simulink subsystem "RoboticArmViperX300"  (R2022a)
settings: Solver=VariableStepAuto  StartTime=0.0  StopTime=10.0  RelTol=1e-3
undefined symbols (not defined in the file or in its folder): smiData, X, Y, Z
libraries: sm_lib x102, nesl_utility x58
(part 1 of 3)
settings Model: Creator=Andy  LastModifiedBy=Andy

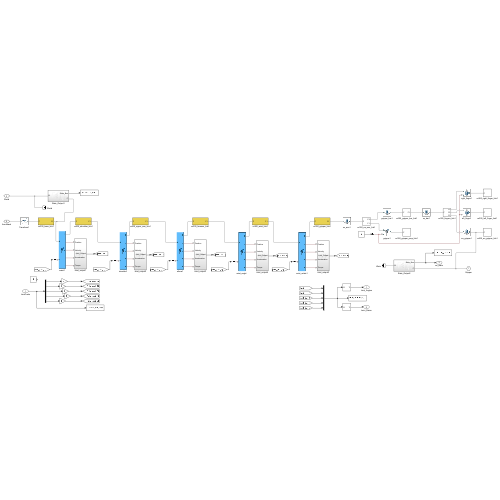
[thumbnail: Simulink's stored preview of the top-level diagram]
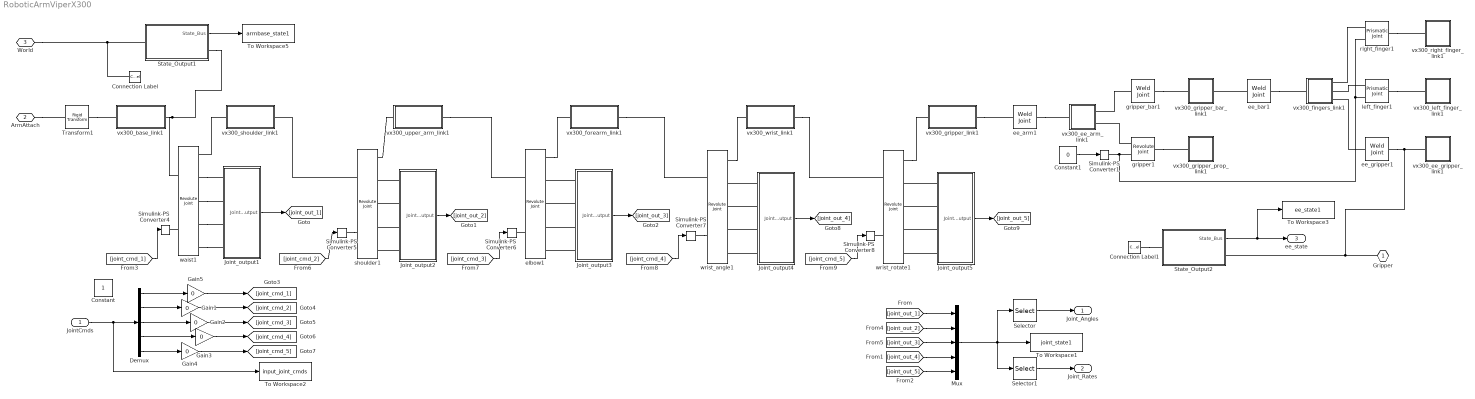
== system RoboticArmViperX300 ==
  JointCmds : Inport
  Connection Label : ConnectionLabel  Label=World
  Connection Label1 : ConnectionLabel  Label=World
  Constant : Constant
  Constant1 : Constant  Value=0
  Demux : Demux  Outputs=5
  Gain{1..5} (5 alike) : Gain  Gain=0
  Joint_output1 : Subsystem
  Joint_output2 : Subsystem
  Joint_output3 : Subsystem
  Joint_output4 : Subsystem
  Joint_output5 : Subsystem
  Mux : Mux  Inputs=5
  Selector : Selector  InputPortWidth=20  IndexOptions=Index vector (dialog)  Indices=[1 5 9 13 17]  OutputSizes=1
  Selector1 : Selector  InputPortWidth=20  IndexOptions=Index vector (dialog)  Indices=[2 6 10 14 18]  OutputSizes=1
  Simulink-PS Converter{1,4..8} (6 alike) : nesl_utility/Simulink-PS Converter  PhysicalDomain=network_engine_domain  SubClassName=ps_input  LeftPortType=input  RightPortType=output  PseudoPeriodic=off  Frequencies=[]  NoiseDistribution=none  NoiseParameters=[]  Unit=1  AffineConversion=off  FilteringAndDerivatives=filter  SimscapeFilterOrder=2  InputFilterTimeConstant=0.001  UdotUserProvided=0
      settings: SourceProductBaseCode=SS,PW,VE
  State_Output1 : Subsystem
  State_Output2 : Subsystem
  To Workspace1 : ToWorkspace  VariableName=joint_state1  SaveFormat=Timeseries  SampleTime=-1
  To Workspace2 : ToWorkspace  VariableName=input_joint_cmds  SaveFormat=Timeseries  SampleTime=-1
  To Workspace3 : ToWorkspace  VariableName=ee_state1  SaveFormat=Timeseries  SampleTime=-1
  To Workspace5 : ToWorkspace  VariableName=armbase_state1  SaveFormat=Timeseries  SampleTime=-1
  Transform1 : sm_lib/Frames and Transforms/Rigid Transform  TranslationMethod=Cartesian  TranslationStandardOffset=0  TranslationLengthUnit=mm  TranslationStandardAxis=+Z  TranslationCartesianOffset=smiData.RigidTransform(1).translation  TranslationROffset=0  TranslationROffsetUnits=m  TranslationZOffset=0  TranslationZOffsetUnits=m  TranslationThetaOffset=0  TranslationThetaOffsetUnits=deg  RotationMethod=ArbitraryAxis  RotationAngleUnits=rad  RotationStandardAxis=+Z  RotationAngle=smiData.RigidTransform(1).angle  RotationArbitraryAxis=smiData.RigidTransform(1).axis  FollAlignAxisA=+X  BaseAlignAxisA=+Y  FollAlignAxisB=+Y  BaseAlignAxisB=+Z  RotationSequenceAxes=FollowerAxes  RotationSequence=YZX  RotationSequenceAngles=[0 0 0]  RotationSequenceAnglesUnits=deg  RotationMatrix=[1 0 0; 0 1 0; 0 0 1]
  ee_arm1 : sm_lib/Joints/Weld Joint  JointMode=Normal  SenseConstraintForce=off  SenseConstraintForceX=off  SenseConstraintForceY=off  SenseConstraintForceZ=off  SenseConstraintTorque=off  SenseConstraintTorqueX=off  SenseConstraintTorqueY=off  SenseConstraintTorqueZ=off  SenseTotalForce=off  SenseTotalForceX=off  SenseTotalForceY=off  SenseTotalForceZ=off  SenseTotalTorque=off  SenseTotalTorqueX=off  SenseTotalTorqueY=off  SenseTotalTorqueZ=off  CompositeWrenchDir=FollowerOnBase  CompositeWrenchFrame=BaseFrame
  ee_bar1 : sm_lib/Joints/Weld Joint  JointMode=Normal  SenseConstraintForce=off  SenseConstraintForceX=off  SenseConstraintForceY=off  SenseConstraintForceZ=off  SenseConstraintTorque=off  SenseConstraintTorqueX=off  SenseConstraintTorqueY=off  SenseConstraintTorqueZ=off  SenseTotalForce=off  SenseTotalForceX=off  SenseTotalForceY=off  SenseTotalForceZ=off  SenseTotalTorque=off  SenseTotalTorqueX=off  SenseTotalTorqueY=off  SenseTotalTorqueZ=off  CompositeWrenchDir=FollowerOnBase  CompositeWrenchFrame=BaseFrame
  ee_gripper1 : sm_lib/Joints/Weld Joint  JointMode=Normal  SenseConstraintForce=off  SenseConstraintForceX=off  SenseConstraintForceY=off  SenseConstraintForceZ=off  SenseConstraintTorque=off  SenseConstraintTorqueX=off  SenseConstraintTorqueY=off  SenseConstraintTorqueZ=off  SenseTotalForce=off  SenseTotalForceX=off  SenseTotalForceY=off  SenseTotalForceZ=off  SenseTotalTorque=off  SenseTotalTorqueX=off  SenseTotalTorqueY=off  SenseTotalTorqueZ=off  CompositeWrenchDir=FollowerOnBase  CompositeWrenchFrame=BaseFrame
  elbow1 : sm_lib/Joints/Revolute Joint  JointMode=Normal  SenseConstraintForce=off  SenseConstraintForceX=off  SenseConstraintForceY=off  SenseConstraintForceZ=off  SenseConstraintTorque=off  SenseConstraintTorqueX=off  SenseConstraintTorqueY=off  SenseConstraintTorqueZ=off  SenseTotalForce=off  SenseTotalForceX=off  SenseTotalForceY=off  SenseTotalForceZ=off  SenseTotalTorque=on  SenseTotalTorqueX=off  SenseTotalTorqueY=off  SenseTotalTorqueZ=off  CompositeWrenchDir=FollowerOnBase  CompositeWrenchFrame=BaseFrame  EquilibriumPosition=0  EquilibriumPositionUnits=deg  SpringStiffness=0  SpringStiffnessUnits=N*m/deg  DampingCoefficient=0  DampingCoefficientUnits=kg*m^2/(rad*s)  TorqueActuationMode=InputTorque  MotionActuationMode=ComputedMotion  SensePosition=on  SenseVelocity=on  SenseAcceleration=on  SenseTorqueForce=off  SenseLowerLimitTorqueForce=off  SenseUpperLimitTorqueForce=off  LowerLimitSpecify=on  LowerLimitBound=-1.762782544514273  LowerLimitBoundUnits=rad  LowerLimitStiffness=1e4  LowerLimitStiffnessUnits=N*m/deg  LowerLimitDamping=10  LowerLimitDampingUnits=N*m/(deg/s)  LowerLimitTransitionRegionWidth=0.1  LowerLimitTransitionRegionWidthUnits=deg  UpperLimitSpecify=on  UpperLimitBound=1.605702911834783  UpperLimitBoundUnits=rad  UpperLimitStiffness=1e4  UpperLimitStiffnessUnits=N*m/deg  UpperLimitDamping=10  UpperLimitDampingUnits=N*m/(deg/s)  UpperLimitTransitionRegionWidth=0.1  UpperLimitTransitionRegionWidthUnits=deg  PositionTargetSpecify=on  PositionTargetPriority=High  PositionTargetValue=smiData.RevoluteJoint(3).Rz.Pos  PositionTargetValueUnits=deg  VelocityTargetSpecify=off  VelocityTargetPriority=High  VelocityTargetValue=0  VelocityTargetValueUnits=deg/s
  gripper1 : sm_lib/Joints/Revolute Joint  JointMode=Normal  SenseConstraintForce=off  SenseConstraintForceX=off  SenseConstraintForceY=off  SenseConstraintForceZ=off  SenseConstraintTorque=off  SenseConstraintTorqueX=off  SenseConstraintTorqueY=off  SenseConstraintTorqueZ=off  SenseTotalForce=off  SenseTotalForceX=off  SenseTotalForceY=off  SenseTotalForceZ=off  SenseTotalTorque=off  SenseTotalTorqueX=off  SenseTotalTorqueY=off  SenseTotalTorqueZ=off  CompositeWrenchDir=FollowerOnBase  CompositeWrenchFrame=BaseFrame  EquilibriumPosition=0  EquilibriumPositionUnits=deg  SpringStiffness=0  SpringStiffnessUnits=N*m/deg  DampingCoefficient=0  DampingCoefficientUnits=kg*m^2/(rad*s)  TorqueActuationMode=ComputedTorque  MotionActuationMode=InputMotion  SensePosition=off  SenseVelocity=off  SenseAcceleration=off  SenseTorqueForce=off  SenseLowerLimitTorqueForce=off  SenseUpperLimitTorqueForce=off  LowerLimitSpecify=off  LowerLimitBound=-90  LowerLimitBoundUnits=deg  LowerLimitStiffness=1e4  LowerLimitStiffnessUnits=N*m/deg  LowerLimitDamping=10  LowerLimitDampingUnits=N*m/(deg/s)  LowerLimitTransitionRegionWidth=0.1  LowerLimitTransitionRegionWidthUnits=deg  UpperLimitSpecify=off  UpperLimitBound=90  UpperLimitBoundUnits=deg  UpperLimitStiffness=1e4  UpperLimitStiffnessUnits=N*m/deg  UpperLimitDamping=10  UpperLimitDampingUnits=N*m/(deg/s)  UpperLimitTransitionRegionWidth=0.1  UpperLimitTransitionRegionWidthUnits=deg  PositionTargetSpecify=off  PositionTargetPriority=High  PositionTargetValue=0  PositionTargetValueUnits=deg  VelocityTargetSpecify=off  VelocityTargetPriority=High  VelocityTargetValue=0  VelocityTargetValueUnits=deg/s
  gripper_bar1 : sm_lib/Joints/Weld Joint  JointMode=Normal  SenseConstraintForce=off  SenseConstraintForceX=off  SenseConstraintForceY=off  SenseConstraintForceZ=off  SenseConstraintTorque=off  SenseConstraintTorqueX=off  SenseConstraintTorqueY=off  SenseConstraintTorqueZ=off  SenseTotalForce=off  SenseTotalForceX=off  SenseTotalForceY=off  SenseTotalForceZ=off  SenseTotalTorque=off  SenseTotalTorqueX=off  SenseTotalTorqueY=off  SenseTotalTorqueZ=off  CompositeWrenchDir=FollowerOnBase  CompositeWrenchFrame=BaseFrame
  left_finger1 : sm_lib/Joints/Prismatic Joint  JointMode=Normal  SenseConstraintForce=off  SenseConstraintForceX=off  SenseConstraintForceY=off  SenseConstraintForceZ=off  SenseConstraintTorque=off  SenseConstraintTorqueX=off  SenseConstraintTorqueY=off  SenseConstraintTorqueZ=off  SenseTotalForce=off  SenseTotalForceX=off  SenseTotalForceY=off  SenseTotalForceZ=off  SenseTotalTorque=off  SenseTotalTorqueX=off  SenseTotalTorqueY=off  SenseTotalTorqueZ=off  CompositeWrenchDir=FollowerOnBase  CompositeWrenchFrame=BaseFrame  EquilibriumPosition=0  EquilibriumPositionUnits=m  SpringStiffness=0  SpringStiffnessUnits=N/m  DampingCoefficient=0  DampingCoefficientUnits=kg/s  TorqueActuationMode=ComputedTorque  MotionActuationMode=InputMotion  SensePosition=off  SenseVelocity=off  SenseAcceleration=off  SenseTorqueForce=off  SenseLowerLimitTorqueForce=off  SenseUpperLimitTorqueForce=off  LowerLimitSpecify=on  LowerLimitBound=0.021  LowerLimitBoundUnits=m  LowerLimitStiffness=1e6  LowerLimitStiffnessUnits=N/m  LowerLimitDamping=1e3  LowerLimitDampingUnits=N/(m/s)  LowerLimitTransitionRegionWidth=1e-4  LowerLimitTransitionRegionWidthUnits=m  UpperLimitSpecify=on  UpperLimitBound=0.057  UpperLimitBoundUnits=m  UpperLimitStiffness=1e6  UpperLimitStiffnessUnits=N/m  UpperLimitDamping=1e3  UpperLimitDampingUnits=N/(m/s)  UpperLimitTransitionRegionWidth=1e-4  UpperLimitTransitionRegionWidthUnits=m  PositionTargetSpecify=off  PositionTargetPriority=High  PositionTargetValue=0  PositionTargetValueUnits=m  VelocityTargetSpecify=off  VelocityTargetPriority=High  VelocityTargetValue=0  VelocityTargetValueUnits=m/s
  right_finger1 : sm_lib/Joints/Prismatic Joint  JointMode=Normal  SenseConstraintForce=off  SenseConstraintForceX=off  SenseConstraintForceY=off  SenseConstraintForceZ=off  SenseConstraintTorque=off  SenseConstraintTorqueX=off  SenseConstraintTorqueY=off  SenseConstraintTorqueZ=off  SenseTotalForce=off  SenseTotalForceX=off  SenseTotalForceY=off  SenseTotalForceZ=off  SenseTotalTorque=off  SenseTotalTorqueX=off  SenseTotalTorqueY=off  SenseTotalTorqueZ=off  CompositeWrenchDir=FollowerOnBase  CompositeWrenchFrame=BaseFrame  EquilibriumPosition=0  EquilibriumPositionUnits=m  SpringStiffness=0  SpringStiffnessUnits=N/m  DampingCoefficient=0  DampingCoefficientUnits=kg/s  TorqueActuationMode=ComputedTorque  MotionActuationMode=InputMotion  SensePosition=off  SenseVelocity=off  SenseAcceleration=off  SenseTorqueForce=off  SenseLowerLimitTorqueForce=off  SenseUpperLimitTorqueForce=off  LowerLimitSpecify=on  LowerLimitBound=-0.057  LowerLimitBoundUnits=m  LowerLimitStiffness=1e6  LowerLimitStiffnessUnits=N/m  LowerLimitDamping=1e3  LowerLimitDampingUnits=N/(m/s)  LowerLimitTransitionRegionWidth=1e-4  LowerLimitTransitionRegionWidthUnits=m  UpperLimitSpecify=on  UpperLimitBound=-0.021  UpperLimitBoundUnits=m  UpperLimitStiffness=1e6  UpperLimitStiffnessUnits=N/m  UpperLimitDamping=1e3  UpperLimitDampingUnits=N/(m/s)  UpperLimitTransitionRegionWidth=1e-4  UpperLimitTransitionRegionWidthUnits=m  PositionTargetSpecify=off  PositionTargetPriority=High  PositionTargetValue=0  PositionTargetValueUnits=m  VelocityTargetSpecify=off  VelocityTargetPriority=High  VelocityTargetValue=0  VelocityTargetValueUnits=m/s
  shoulder1 : sm_lib/Joints/Revolute Joint  JointMode=Normal  SenseConstraintForce=off  SenseConstraintForceX=off  SenseConstraintForceY=off  SenseConstraintForceZ=off  SenseConstraintTorque=off  SenseConstraintTorqueX=off  SenseConstraintTorqueY=off  SenseConstraintTorqueZ=off  SenseTotalForce=off  SenseTotalForceX=off  SenseTotalForceY=off  SenseTotalForceZ=off  SenseTotalTorque=on  SenseTotalTorqueX=off  SenseTotalTorqueY=off  SenseTotalTorqueZ=off  CompositeWrenchDir=FollowerOnBase  CompositeWrenchFrame=BaseFrame  EquilibriumPosition=0  EquilibriumPositionUnits=deg  SpringStiffness=0  SpringStiffnessUnits=N*m/deg  DampingCoefficient=0  DampingCoefficientUnits=kg*m^2/(rad*s)  TorqueActuationMode=InputTorque  MotionActuationMode=ComputedMotion  SensePosition=on  SenseVelocity=on  SenseAcceleration=on  SenseTorqueForce=off  SenseLowerLimitTorqueForce=off  SenseUpperLimitTorqueForce=off  LowerLimitSpecify=on  LowerLimitBound=-1.850049007113989  LowerLimitBoundUnits=rad  LowerLimitStiffness=1e4  LowerLimitStiffnessUnits=N*m/deg  LowerLimitDamping=10  LowerLimitDampingUnits=N*m/(deg/s)  LowerLimitTransitionRegionWidth=0.1  LowerLimitTransitionRegionWidthUnits=deg  UpperLimitSpecify=on  UpperLimitBound=1.256637061435917  UpperLimitBoundUnits=rad  UpperLimitStiffness=1e4  UpperLimitStiffnessUnits=N*m/deg  UpperLimitDamping=10  UpperLimitDampingUnits=N*m/(deg/s)  UpperLimitTransitionRegionWidth=0.1  UpperLimitTransitionRegionWidthUnits=deg  PositionTargetSpecify=on  PositionTargetPriority=High  PositionTargetValue=smiData.RevoluteJoint(2).Rz.Pos  PositionTargetValueUnits=deg  VelocityTargetSpecify=off  VelocityTargetPriority=High  VelocityTargetValue=0  VelocityTargetValueUnits=deg/s
  vx300_base_link1 : Subsystem
  vx300_ee_arm_link1 : Subsystem
  vx300_ee_gripper_link1 : Subsystem
  vx300_fingers_link1 : Subsystem
  vx300_forearm_link1 : Subsystem
  vx300_gripper_bar_link1 : Subsystem
  vx300_gripper_link1 : Subsystem
  vx300_gripper_prop_link1 : Subsystem
  vx300_left_finger_link1 : Subsystem
  vx300_right_finger_link1 : Subsystem
  vx300_shoulder_link1 : Subsystem
  vx300_upper_arm_link1 : Subsystem
  vx300_wrist_link1 : Subsystem
  waist1 : sm_lib/Joints/Revolute Joint  JointMode=Normal  SenseConstraintForce=off  SenseConstraintForceX=off  SenseConstraintForceY=off  SenseConstraintForceZ=off  SenseConstraintTorque=off  SenseConstraintTorqueX=off  SenseConstraintTorqueY=off  SenseConstraintTorqueZ=off  SenseTotalForce=off  SenseTotalForceX=off  SenseTotalForceY=off  SenseTotalForceZ=off  SenseTotalTorque=on  SenseTotalTorqueX=off  SenseTotalTorqueY=off  SenseTotalTorqueZ=off  CompositeWrenchDir=FollowerOnBase  CompositeWrenchFrame=BaseFrame  EquilibriumPosition=0  EquilibriumPositionUnits=deg  SpringStiffness=0  SpringStiffnessUnits=N*m/deg  DampingCoefficient=0  DampingCoefficientUnits=kg*m^2/(rad*s)  TorqueActuationMode=InputTorque  MotionActuationMode=ComputedMotion  SensePosition=on  SenseVelocity=on  SenseAcceleration=on  SenseTorqueForce=off  SenseLowerLimitTorqueForce=off  SenseUpperLimitTorqueForce=off  LowerLimitSpecify=on  LowerLimitBound=-3.141582653589793  LowerLimitBoundUnits=rad  LowerLimitStiffness=1e4  LowerLimitStiffnessUnits=N*m/deg  LowerLimitDamping=10  LowerLimitDampingUnits=N*m/(deg/s)  LowerLimitTransitionRegionWidth=0.1  LowerLimitTransitionRegionWidthUnits=deg  UpperLimitSpecify=on  UpperLimitBound=3.141582653589793  UpperLimitBoundUnits=rad  UpperLimitStiffness=1e4  UpperLimitStiffnessUnits=N*m/deg  UpperLimitDamping=10  UpperLimitDampingUnits=N*m/(deg/s)  UpperLimitTransitionRegionWidth=0.1  UpperLimitTransitionRegionWidthUnits=deg  PositionTargetSpecify=on  PositionTargetPriority=High  PositionTargetValue=smiData.RevoluteJoint(1).Rz.Pos  PositionTargetValueUnits=deg  VelocityTargetSpecify=off  VelocityTargetPriority=High  VelocityTargetValue=0  VelocityTargetValueUnits=deg/s
  wrist_angle1 : sm_lib/Joints/Revolute Joint  JointMode=Normal  SenseConstraintForce=off  SenseConstraintForceX=off  SenseConstraintForceY=off  SenseConstraintForceZ=off  SenseConstraintTorque=off  SenseConstraintTorqueX=off  SenseConstraintTorqueY=off  SenseConstraintTorqueZ=off  SenseTotalForce=off  SenseTotalForceX=off  SenseTotalForceY=off  SenseTotalForceZ=off  SenseTotalTorque=on  SenseTotalTorqueX=off  SenseTotalTorqueY=off  SenseTotalTorqueZ=off  CompositeWrenchDir=FollowerOnBase  CompositeWrenchFrame=BaseFrame  EquilibriumPosition=0  EquilibriumPositionUnits=deg  SpringStiffness=0  SpringStiffnessUnits=N*m/deg  DampingCoefficient=0  DampingCoefficientUnits=kg*m^2/(rad*s)  TorqueActuationMode=InputTorque  MotionActuationMode=ComputedMotion  SensePosition=on  SenseVelocity=on  SenseAcceleration=on  SenseTorqueForce=off  SenseLowerLimitTorqueForce=off  SenseUpperLimitTorqueForce=off  LowerLimitSpecify=on  LowerLimitBound=-1.867502299633933  LowerLimitBoundUnits=rad  LowerLimitStiffness=1e4  LowerLimitStiffnessUnits=N*m/deg  LowerLimitDamping=10  LowerLimitDampingUnits=N*m/(deg/s)  LowerLimitTransitionRegionWidth=0.1  LowerLimitTransitionRegionWidthUnits=deg  UpperLimitSpecify=on  UpperLimitBound=2.234021442552742  UpperLimitBoundUnits=rad  UpperLimitStiffness=1e4  UpperLimitStiffnessUnits=N*m/deg  UpperLimitDamping=10  UpperLimitDampingUnits=N*m/(deg/s)  UpperLimitTransitionRegionWidth=0.1  UpperLimitTransitionRegionWidthUnits=deg  PositionTargetSpecify=on  PositionTargetPriority=High  PositionTargetValue=smiData.RevoluteJoint(4).Rz.Pos  PositionTargetValueUnits=deg  VelocityTargetSpecify=off  VelocityTargetPriority=High  VelocityTargetValue=0  VelocityTargetValueUnits=deg/s
  wrist_rotate1 : sm_lib/Joints/Revolute Joint  JointMode=Normal  SenseConstraintForce=off  SenseConstraintForceX=off  SenseConstraintForceY=off  SenseConstraintForceZ=off  SenseConstraintTorque=off  SenseConstraintTorqueX=off  SenseConstraintTorqueY=off  SenseConstraintTorqueZ=off  SenseTotalForce=off  SenseTotalForceX=off  SenseTotalForceY=off  SenseTotalForceZ=off  SenseTotalTorque=on  SenseTotalTorqueX=off  SenseTotalTorqueY=off  SenseTotalTorqueZ=off  CompositeWrenchDir=FollowerOnBase  CompositeWrenchFrame=BaseFrame  EquilibriumPosition=0  EquilibriumPositionUnits=deg  SpringStiffness=0  SpringStiffnessUnits=N*m/deg  DampingCoefficient=0  DampingCoefficientUnits=kg*m^2/(rad*s)  TorqueActuationMode=InputTorque  MotionActuationMode=ComputedMotion  SensePosition=on  SenseVelocity=on  SenseAcceleration=on  SenseTorqueForce=off  SenseLowerLimitTorqueForce=off  SenseUpperLimitTorqueForce=off  LowerLimitSpecify=on  LowerLimitBound=-3.141582653589793  LowerLimitBoundUnits=rad  LowerLimitStiffness=1e4  LowerLimitStiffnessUnits=N*m/deg  LowerLimitDamping=10  LowerLimitDampingUnits=N*m/(deg/s)  LowerLimitTransitionRegionWidth=0.1  LowerLimitTransitionRegionWidthUnits=deg  UpperLimitSpecify=on  UpperLimitBound=3.141582653589793  UpperLimitBoundUnits=rad  UpperLimitStiffness=1e4  UpperLimitStiffnessUnits=N*m/deg  UpperLimitDamping=10  UpperLimitDampingUnits=N*m/(deg/s)  UpperLimitTransitionRegionWidth=0.1  UpperLimitTransitionRegionWidthUnits=deg  PositionTargetSpecify=on  PositionTargetPriority=High  PositionTargetValue=smiData.RevoluteJoint(5).Rz.Pos  PositionTargetValueUnits=deg  VelocityTargetSpecify=off  VelocityTargetPriority=High  VelocityTargetValue=0  VelocityTargetValueUnits=deg/s
  Gripper : PMIOPort  Side=Right
  ArmAttach : PMIOPort  Port=2  Side=Left
  World : PMIOPort  Port=3  Side=Left
  Joint_Angles : Outport
  Joint_Rates : Outport  Port=2
  ee_state : Outport  Port=3
  wires:
  Joint_output3/1(Joint_Output) -> [joint_out_3]
  [joint_out_1] -> Mux/1
  Selector/1 -> Joint_Angles/1
  JointCmds/1 -> Demux/1, To Workspace2/1
  State_Output2/1(State_Bus) -> ee_state/1, To Workspace3/1
  State_Output1/1(State_Bus) -> To Workspace5/1
  Joint_output1/1(Joint_Output) -> [joint_out_1]
  Demux/2 -> Gain1/1
  Demux/3 -> Gain2/1
  Demux/4 -> Gain3/1
  Demux/5 -> Gain4/1
  [joint_cmd_1] -> Simulink-PS Converter4/1
  [joint_cmd_2] -> Simulink-PS Converter5/1
  Joint_output2/1(Joint_Output) -> [joint_out_2]
  [joint_cmd_3] -> Simulink-PS Converter6/1
  Joint_output4/1(Joint_Output) -> [joint_out_4]
  [joint_cmd_4] -> Simulink-PS Converter7/1
  [joint_cmd_5] -> Simulink-PS Converter8/1
  Joint_output5/1(Joint_Output) -> [joint_out_5]
  Mux/1 -> Selector1/1, To Workspace1/1, Selector/1
  Selector1/1 -> Joint_Rates/1
  Gain5/1 -> [joint_cmd_1]
  Gain1/1 -> [joint_cmd_2]
  Gain2/1 -> [joint_cmd_3]
  Gain3/1 -> [joint_cmd_4]
  Gain4/1 -> [joint_cmd_5]
  Demux/1 -> Gain5/1
  [joint_out_2] -> Mux/2
  [joint_out_3] -> Mux/3
  [joint_out_4] -> Mux/4
  [joint_out_5] -> Mux/5
  Constant1/1 -> Simulink-PS Converter1/1
  connections:
  World/RConn1 -- Connection Label/LConn1 -- State_Output1/LConn1
  vx300_base_link1/RConn1 -- State_Output1/RConn1 -- waist1/LConn1
  Connection Label1/LConn1 -- State_Output2/LConn1
  right_finger1/LConn1 -- vx300_fingers_link1/RConn1
  left_finger1/LConn1 -- vx300_fingers_link1/RConn2
  shoulder1/LConn1 -- vx300_shoulder_link1/RConn1
  Gripper/RConn1 -- vx300_ee_gripper_link1/LConn1 -- ee_gripper1/RConn1 -- State_Output2/RConn1
  elbow1/RConn1 -- vx300_forearm_link1/LConn1
  vx300_upper_arm_link1/RConn1 -- elbow1/LConn1
  gripper1/LConn1 -- vx300_ee_arm_link1/RConn2
  gripper1/RConn1 -- vx300_gripper_prop_link1/LConn1
  ee_arm1/RConn1 -- vx300_ee_arm_link1/LConn1
  ee_bar1/RConn1 -- vx300_fingers_link1/LConn1
  ee_bar1/LConn1 -- vx300_gripper_bar_link1/RConn1
  gripper_bar1/LConn1 -- vx300_ee_arm_link1/RConn1
  gripper_bar1/RConn1 -- vx300_gripper_bar_link1/LConn1
  vx300_forearm_link1/RConn1 -- wrist_angle1/LConn1
  vx300_wrist_link1/RConn1 -- wrist_rotate1/LConn1
  right_finger1/RConn1 -- vx300_right_finger_link1/LConn1
  left_finger1/RConn1 -- vx300_left_finger_link1/LConn1
  vx300_gripper_link1/RConn1 -- ee_arm1/LConn1
  wrist_angle1/RConn1 -- vx300_wrist_link1/LConn1
  Simulink-PS Converter4/RConn1 -- waist1/LConn2
  waist1/RConn2 -- Joint_output1/LConn1
  waist1/RConn3 -- Joint_output1/LConn2
  waist1/RConn4 -- Joint_output1/LConn3
  waist1/RConn5 -- Joint_output1/LConn4
  Simulink-PS Converter5/RConn1 -- shoulder1/LConn2
  Joint_output2/LConn3 -- shoulder1/RConn4
  Joint_output2/LConn2 -- shoulder1/RConn3
  Joint_output2/LConn4 -- shoulder1/RConn5
  Joint_output2/LConn1 -- shoulder1/RConn2
  Joint_output3/LConn1 -- elbow1/RConn2
  Joint_output3/LConn2 -- elbow1/RConn3
  Joint_output3/LConn3 -- elbow1/RConn4
  Joint_output3/LConn4 -- elbow1/RConn5
  Simulink-PS Converter6/RConn1 -- elbow1/LConn2
  Joint_output4/LConn1 -- wrist_angle1/RConn2
  Joint_output4/LConn2 -- wrist_angle1/RConn3
  Joint_output4/LConn3 -- wrist_angle1/RConn4
  Joint_output4/LConn4 -- wrist_angle1/RConn5
  Simulink-PS Converter7/RConn1 -- wrist_angle1/LConn2
  wrist_rotate1/LConn2 -- Simulink-PS Converter8/RConn1
  Joint_output5/LConn1 -- wrist_rotate1/RConn2
  Joint_output5/LConn2 -- wrist_rotate1/RConn3
  Joint_output5/LConn3 -- wrist_rotate1/RConn4
  Joint_output5/LConn4 -- wrist_rotate1/RConn5
  Transform1/RConn1 -- vx300_base_link1/LConn1
  ArmAttach/RConn1 -- Transform1/LConn1
  ee_gripper1/LConn1 -- vx300_fingers_link1/RConn3
  wrist_rotate1/RConn1 -- vx300_gripper_link1/LConn1
  vx300_shoulder_link1/LConn1 -- waist1/RConn1
  vx300_upper_arm_link1/LConn1 -- shoulder1/RConn1
  Simulink-PS Converter1/RConn1 -- right_finger1/LConn2 -- left_finger1/LConn2 -- gripper1/LConn2

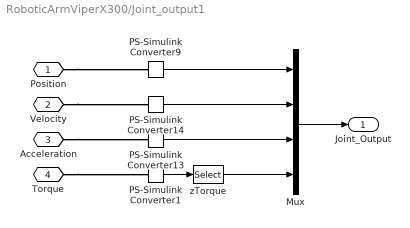
== system RoboticArmViperX300/Joint_output1 ==
  Mux : Mux
  PS-Simulink Converter{1,9,13..14} (4 alike) : nesl_utility/PS-Simulink Converter  PhysicalDomain=network_engine_domain  SubClassName=ps_output  LeftPortType=input  RightPortType=output  PseudoPeriodic=off  Frequencies=[]  VectorFormat=1-D array  Unit=inherit  AffineConversion=off
      settings: SourceProductBaseCode=SS,PW,VE
  zTorque : Selector  InputPortWidth=3  IndexOptions=Index vector (dialog)  Indices=3  OutputSizes=1
  Position : PMIOPort  Side=Left
  Velocity : PMIOPort  Port=2  Side=Left
  Acceleration : PMIOPort  Port=3  Side=Left
  Torque : PMIOPort  Port=4  Side=Left
  Joint_Output : Outport
  wires:
  zTorque/1 -> Mux/4
  PS-Simulink Converter1/1 -> zTorque/1
  PS-Simulink Converter13/1 -> Mux/3
  PS-Simulink Converter14/1 -> Mux/2
  PS-Simulink Converter9/1 -> Mux/1
  Mux/1 -> Joint_Output/1
  connections:
  Torque/RConn1 -- PS-Simulink Converter1/LConn1
  Position/RConn1 -- PS-Simulink Converter9/LConn1
  Acceleration/RConn1 -- PS-Simulink Converter13/LConn1
  Velocity/RConn1 -- PS-Simulink Converter14/LConn1

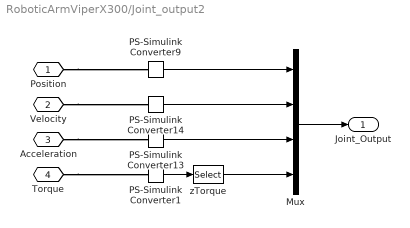
== system RoboticArmViperX300/Joint_output2 ==
  Mux : Mux
  PS-Simulink Converter{1,9,13..14} (4 alike) : nesl_utility/PS-Simulink Converter  PhysicalDomain=network_engine_domain  SubClassName=ps_output  LeftPortType=input  RightPortType=output  PseudoPeriodic=off  Frequencies=[]  VectorFormat=1-D array  Unit=inherit  AffineConversion=off
      settings: SourceProductBaseCode=SS,PW,VE
  zTorque : Selector  InputPortWidth=3  IndexOptions=Index vector (dialog)  Indices=3  OutputSizes=1
  Position : PMIOPort  Side=Left
  Velocity : PMIOPort  Port=2  Side=Left
  Acceleration : PMIOPort  Port=3  Side=Left
  Torque : PMIOPort  Port=4  Side=Left
  Joint_Output : Outport
  wires:
  zTorque/1 -> Mux/4
  PS-Simulink Converter1/1 -> zTorque/1
  PS-Simulink Converter13/1 -> Mux/3
  PS-Simulink Converter14/1 -> Mux/2
  PS-Simulink Converter9/1 -> Mux/1
  Mux/1 -> Joint_Output/1
  connections:
  Torque/RConn1 -- PS-Simulink Converter1/LConn1
  Position/RConn1 -- PS-Simulink Converter9/LConn1
  Acceleration/RConn1 -- PS-Simulink Converter13/LConn1
  Velocity/RConn1 -- PS-Simulink Converter14/LConn1

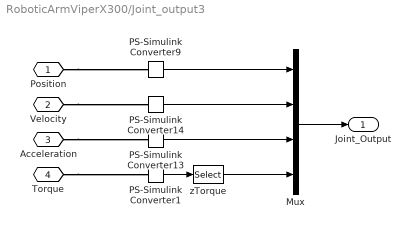
== system RoboticArmViperX300/Joint_output3 ==
  Mux : Mux
  PS-Simulink Converter{1,9,13..14} (4 alike) : nesl_utility/PS-Simulink Converter  PhysicalDomain=network_engine_domain  SubClassName=ps_output  LeftPortType=input  RightPortType=output  PseudoPeriodic=off  Frequencies=[]  VectorFormat=1-D array  Unit=inherit  AffineConversion=off
      settings: SourceProductBaseCode=SS,PW,VE
  zTorque : Selector  InputPortWidth=3  IndexOptions=Index vector (dialog)  Indices=3  OutputSizes=1
  Position : PMIOPort  Side=Left
  Velocity : PMIOPort  Port=2  Side=Left
  Acceleration : PMIOPort  Port=3  Side=Left
  Torque : PMIOPort  Port=4  Side=Left
  Joint_Output : Outport
  wires:
  zTorque/1 -> Mux/4
  PS-Simulink Converter1/1 -> zTorque/1
  PS-Simulink Converter13/1 -> Mux/3
  PS-Simulink Converter14/1 -> Mux/2
  PS-Simulink Converter9/1 -> Mux/1
  Mux/1 -> Joint_Output/1
  connections:
  Torque/RConn1 -- PS-Simulink Converter1/LConn1
  Position/RConn1 -- PS-Simulink Converter9/LConn1
  Acceleration/RConn1 -- PS-Simulink Converter13/LConn1
  Velocity/RConn1 -- PS-Simulink Converter14/LConn1

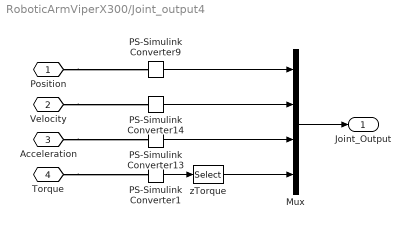
== system RoboticArmViperX300/Joint_output4 ==
  Mux : Mux
  PS-Simulink Converter{1,9,13..14} (4 alike) : nesl_utility/PS-Simulink Converter  PhysicalDomain=network_engine_domain  SubClassName=ps_output  LeftPortType=input  RightPortType=output  PseudoPeriodic=off  Frequencies=[]  VectorFormat=1-D array  Unit=inherit  AffineConversion=off
      settings: SourceProductBaseCode=SS,PW,VE
  zTorque : Selector  InputPortWidth=3  IndexOptions=Index vector (dialog)  Indices=3  OutputSizes=1
  Position : PMIOPort  Side=Left
  Velocity : PMIOPort  Port=2  Side=Left
  Acceleration : PMIOPort  Port=3  Side=Left
  Torque : PMIOPort  Port=4  Side=Left
  Joint_Output : Outport
  wires:
  zTorque/1 -> Mux/4
  PS-Simulink Converter1/1 -> zTorque/1
  PS-Simulink Converter13/1 -> Mux/3
  PS-Simulink Converter14/1 -> Mux/2
  PS-Simulink Converter9/1 -> Mux/1
  Mux/1 -> Joint_Output/1
  connections:
  Torque/RConn1 -- PS-Simulink Converter1/LConn1
  Position/RConn1 -- PS-Simulink Converter9/LConn1
  Acceleration/RConn1 -- PS-Simulink Converter13/LConn1
  Velocity/RConn1 -- PS-Simulink Converter14/LConn1

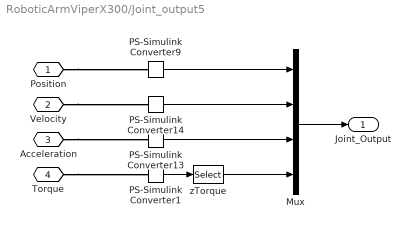
== system RoboticArmViperX300/Joint_output5 ==
  Mux : Mux
  PS-Simulink Converter{1,9,13..14} (4 alike) : nesl_utility/PS-Simulink Converter  PhysicalDomain=network_engine_domain  SubClassName=ps_output  LeftPortType=input  RightPortType=output  PseudoPeriodic=off  Frequencies=[]  VectorFormat=1-D array  Unit=inherit  AffineConversion=off
      settings: SourceProductBaseCode=SS,PW,VE
  zTorque : Selector  InputPortWidth=3  IndexOptions=Index vector (dialog)  Indices=3  OutputSizes=1
  Position : PMIOPort  Side=Left
  Velocity : PMIOPort  Port=2  Side=Left
  Acceleration : PMIOPort  Port=3  Side=Left
  Torque : PMIOPort  Port=4  Side=Left
  Joint_Output : Outport
  wires:
  zTorque/1 -> Mux/4
  PS-Simulink Converter1/1 -> zTorque/1
  PS-Simulink Converter13/1 -> Mux/3
  PS-Simulink Converter14/1 -> Mux/2
  PS-Simulink Converter9/1 -> Mux/1
  Mux/1 -> Joint_Output/1
  connections:
  Torque/RConn1 -- PS-Simulink Converter1/LConn1
  Position/RConn1 -- PS-Simulink Converter9/LConn1
  Acceleration/RConn1 -- PS-Simulink Converter13/LConn1
  Velocity/RConn1 -- PS-Simulink Converter14/LConn1

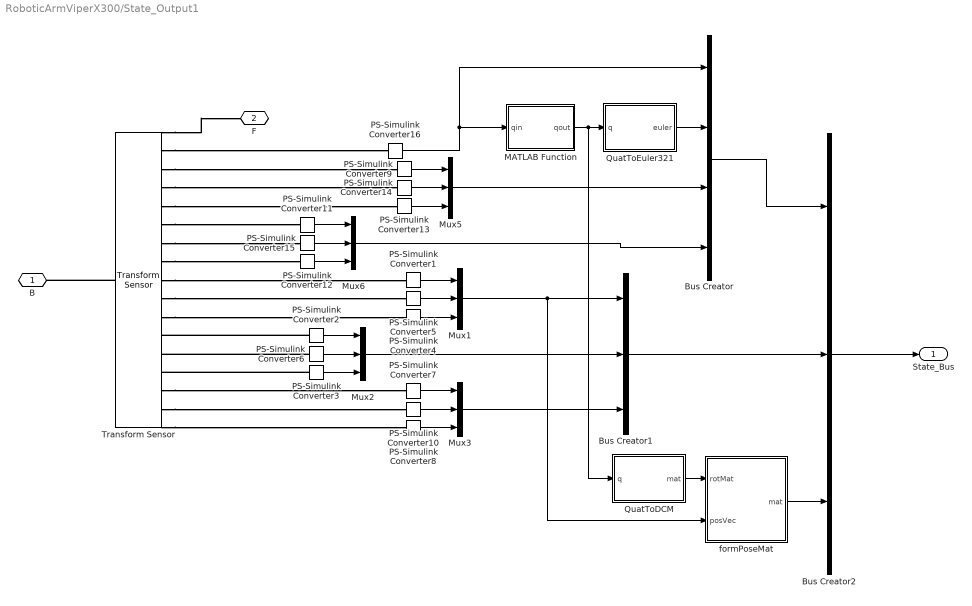
== system RoboticArmViperX300/State_Output1 ==
  Bus Creator : BusCreator  Inputs=4  OutDataTypeStr=Bus: RotStateBus
      settings: InheritFromInputs=off
  Bus Creator1 : BusCreator  Inputs=3  OutDataTypeStr=Bus: TransStateBus
      settings: InheritFromInputs=off
  Bus Creator2 : BusCreator  Inputs=3  OutDataTypeStr=Bus: StateBus
      settings: InheritFromInputs=off
  MATLAB Function : MATLAB Function  TreatAsAtomicUnit=on
  Mux{1..3,5..6} (5 alike) : Mux  Inputs=3
  PS-Simulink Converter{1..16} (16 alike) : nesl_utility/PS-Simulink Converter  PhysicalDomain=network_engine_domain  SubClassName=ps_output  LeftPortType=input  RightPortType=output  PseudoPeriodic=off  Frequencies=[]  VectorFormat=1-D array  Unit=inherit  AffineConversion=off
      settings: SourceProductBaseCode=SS,PW,VE
  QuatToDCM : MATLAB Function  TreatAsAtomicUnit=on
  QuatToEuler321 : MATLAB Function  TreatAsAtomicUnit=on
  Transform Sensor : sm_lib/Frames and Transforms/Transform Sensor  MeasurementFrame=World  SenseAngle=off  SenseAxis=off  SenseAngle1=off  SenseAngle2=off  SenseAngle3=off  SenseQ=on  SenseR=off  SenseOmegaX=on  SenseOmegaY=on  SenseOmegaZ=on  SenseOmega1=off  SenseOmega2=off  SenseOmega3=off  SenseQDot=off  SenseRDot=off  SenseAlphaX=on  SenseAlphaY=on  SenseAlphaZ=on  SenseAlpha1=off  SenseAlpha2=off  SenseAlpha3=off  SenseQDDot=off  SenseRDDot=off  SenseX=on  SenseY=on  SenseZ=on  SenseRad=off  SenseAzim=off  SenseDist=off  SenseInc=off  SenseXDot=on  SenseYDot=on  SenseZDot=on  SenseRadDot=off  SenseAzimDot=off  SenseDistDot=off  SenseIncDot=off  SenseXDDot=on  SenseYDDot=on  SenseZDDot=on  SenseRadDDot=off  SenseAzimDDot=off  SenseDistDDot=off  SenseIncDDot=off
  formPoseMat : MATLAB Function  TreatAsAtomicUnit=on
  B : PMIOPort  Side=Left
  F : PMIOPort  Port=2  Side=Right
  State_Bus : Outport
  wires:
  formPoseMat/1(mat) -> Bus Creator2/3
  QuatToDCM/1(mat) -> formPoseMat/1(rotMat)
  MATLAB Function/1(qout) -> QuatToEuler321/1(q), QuatToDCM/1(q)
  Bus Creator2/1 -> State_Bus/1
  Bus Creator1/1 -> Bus Creator2/2
  Bus Creator/1 -> Bus Creator2/1
  QuatToEuler321/1(euler) -> Bus Creator/2
  PS-Simulink Converter16/1 -> MATLAB Function/1(qin), Bus Creator/1
  PS-Simulink Converter11/1 -> Mux6/1
  Mux6/1 -> Bus Creator/4
  PS-Simulink Converter12/1 -> Mux6/3
  PS-Simulink Converter15/1 -> Mux6/2
  Mux5/1 -> Bus Creator/3
  PS-Simulink Converter13/1 -> Mux5/3
  PS-Simulink Converter14/1 -> Mux5/2
  PS-Simulink Converter9/1 -> Mux5/1
  Mux3/1 -> Bus Creator1/3
  Mux1/1 -> Bus Creator1/1, formPoseMat/2(posVec)
  Mux2/1 -> Bus Creator1/2
  PS-Simulink Converter7/1 -> Mux3/1
  PS-Simulink Converter8/1 -> Mux3/3
  PS-Simulink Converter10/1 -> Mux3/2
  PS-Simulink Converter2/1 -> Mux2/1
  PS-Simulink Converter6/1 -> Mux2/2
  PS-Simulink Converter3/1 -> Mux2/3
  PS-Simulink Converter1/1 -> Mux1/1
  PS-Simulink Converter5/1 -> Mux1/2
  PS-Simulink Converter4/1 -> Mux1/3
  connections:
  Transform Sensor/RConn2 -- PS-Simulink Converter16/LConn1
  Transform Sensor/RConn6 -- PS-Simulink Converter11/LConn1
  Transform Sensor/RConn7 -- PS-Simulink Converter15/LConn1
  Transform Sensor/RConn3 -- PS-Simulink Converter9/LConn1
  Transform Sensor/RConn4 -- PS-Simulink Converter14/LConn1
  Transform Sensor/RConn5 -- PS-Simulink Converter13/LConn1
  Transform Sensor/RConn8 -- PS-Simulink Converter12/LConn1
  Transform Sensor/RConn16 -- PS-Simulink Converter10/LConn1
  Transform Sensor/RConn15 -- PS-Simulink Converter7/LConn1
  Transform Sensor/RConn17 -- PS-Simulink Converter8/LConn1
  PS-Simulink Converter2/LConn1 -- Transform Sensor/RConn12
  PS-Simulink Converter6/LConn1 -- Transform Sensor/RConn13
  PS-Simulink Converter3/LConn1 -- Transform Sensor/RConn14
  Transform Sensor/RConn11 -- PS-Simulink Converter4/LConn1
  Transform Sensor/RConn10 -- PS-Simulink Converter5/LConn1
  Transform Sensor/RConn9 -- PS-Simulink Converter1/LConn1
  Transform Sensor/RConn1 -- F/RConn1
  Transform Sensor/LConn1 -- B/RConn1

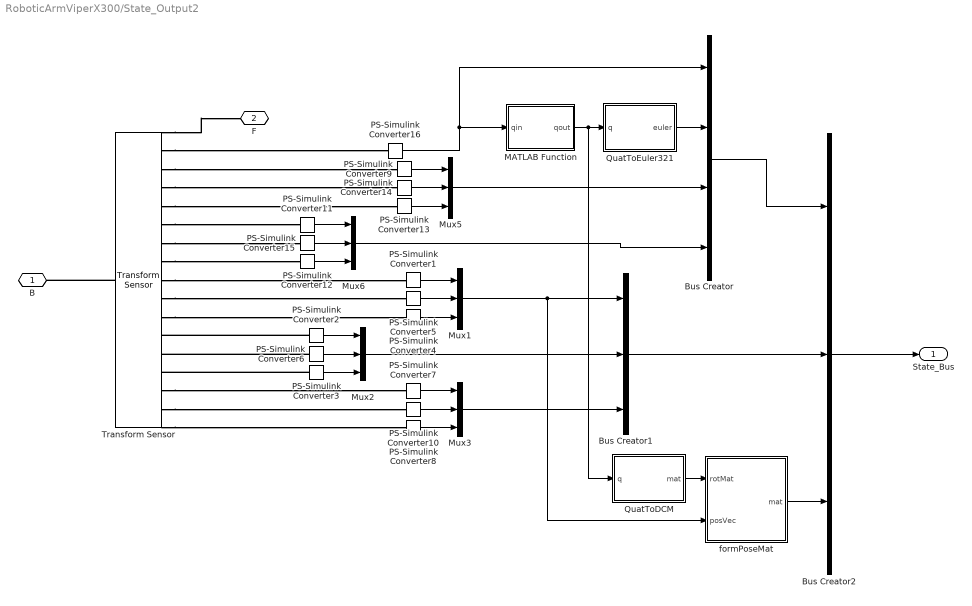
== system RoboticArmViperX300/State_Output2 ==
  Bus Creator : BusCreator  Inputs=4  OutDataTypeStr=Bus: RotStateBus
      settings: InheritFromInputs=off
  Bus Creator1 : BusCreator  Inputs=3  OutDataTypeStr=Bus: TransStateBus
      settings: InheritFromInputs=off
  Bus Creator2 : BusCreator  Inputs=3  OutDataTypeStr=Bus: StateBus
      settings: InheritFromInputs=off
  MATLAB Function : MATLAB Function  TreatAsAtomicUnit=on
  Mux{1..3,5..6} (5 alike) : Mux  Inputs=3
  PS-Simulink Converter{1..16} (16 alike) : nesl_utility/PS-Simulink Converter  PhysicalDomain=network_engine_domain  SubClassName=ps_output  LeftPortType=input  RightPortType=output  PseudoPeriodic=off  Frequencies=[]  VectorFormat=1-D array  Unit=inherit  AffineConversion=off
      settings: SourceProductBaseCode=SS,PW,VE
  QuatToDCM : MATLAB Function  TreatAsAtomicUnit=on
  QuatToEuler321 : MATLAB Function  TreatAsAtomicUnit=on
  Transform Sensor : sm_lib/Frames and Transforms/Transform Sensor  MeasurementFrame=World  SenseAngle=off  SenseAxis=off  SenseAngle1=off  SenseAngle2=off  SenseAngle3=off  SenseQ=on  SenseR=off  SenseOmegaX=on  SenseOmegaY=on  SenseOmegaZ=on  SenseOmega1=off  SenseOmega2=off  SenseOmega3=off  SenseQDot=off  SenseRDot=off  SenseAlphaX=on  SenseAlphaY=on  SenseAlphaZ=on  SenseAlpha1=off  SenseAlpha2=off  SenseAlpha3=off  SenseQDDot=off  SenseRDDot=off  SenseX=on  SenseY=on  SenseZ=on  SenseRad=off  SenseAzim=off  SenseDist=off  SenseInc=off  SenseXDot=on  SenseYDot=on  SenseZDot=on  SenseRadDot=off  SenseAzimDot=off  SenseDistDot=off  SenseIncDot=off  SenseXDDot=on  SenseYDDot=on  SenseZDDot=on  SenseRadDDot=off  SenseAzimDDot=off  SenseDistDDot=off  SenseIncDDot=off
  formPoseMat : MATLAB Function  TreatAsAtomicUnit=on
  B : PMIOPort  Side=Left
  F : PMIOPort  Port=2  Side=Right
  State_Bus : Outport
  wires:
  formPoseMat/1(mat) -> Bus Creator2/3
  QuatToDCM/1(mat) -> formPoseMat/1(rotMat)
  MATLAB Function/1(qout) -> QuatToEuler321/1(q), QuatToDCM/1(q)
  Bus Creator2/1 -> State_Bus/1
  Bus Creator1/1 -> Bus Creator2/2
  Bus Creator/1 -> Bus Creator2/1
  QuatToEuler321/1(euler) -> Bus Creator/2
  PS-Simulink Converter16/1 -> MATLAB Function/1(qin), Bus Creator/1
  PS-Simulink Converter11/1 -> Mux6/1
  Mux6/1 -> Bus Creator/4
  PS-Simulink Converter12/1 -> Mux6/3
  PS-Simulink Converter15/1 -> Mux6/2
  Mux5/1 -> Bus Creator/3
  PS-Simulink Converter13/1 -> Mux5/3
  PS-Simulink Converter14/1 -> Mux5/2
  PS-Simulink Converter9/1 -> Mux5/1
  Mux3/1 -> Bus Creator1/3
  Mux1/1 -> Bus Creator1/1, formPoseMat/2(posVec)
  Mux2/1 -> Bus Creator1/2
  PS-Simulink Converter7/1 -> Mux3/1
  PS-Simulink Converter8/1 -> Mux3/3
  PS-Simulink Converter10/1 -> Mux3/2
  PS-Simulink Converter2/1 -> Mux2/1
  PS-Simulink Converter6/1 -> Mux2/2
  PS-Simulink Converter3/1 -> Mux2/3
  PS-Simulink Converter1/1 -> Mux1/1
  PS-Simulink Converter5/1 -> Mux1/2
  PS-Simulink Converter4/1 -> Mux1/3
  connections:
  Transform Sensor/RConn2 -- PS-Simulink Converter16/LConn1
  Transform Sensor/RConn6 -- PS-Simulink Converter11/LConn1
  Transform Sensor/RConn7 -- PS-Simulink Converter15/LConn1
  Transform Sensor/RConn3 -- PS-Simulink Converter9/LConn1
  Transform Sensor/RConn4 -- PS-Simulink Converter14/LConn1
  Transform Sensor/RConn5 -- PS-Simulink Converter13/LConn1
  Transform Sensor/RConn8 -- PS-Simulink Converter12/LConn1
  Transform Sensor/RConn16 -- PS-Simulink Converter10/LConn1
  Transform Sensor/RConn15 -- PS-Simulink Converter7/LConn1
  Transform Sensor/RConn17 -- PS-Simulink Converter8/LConn1
  PS-Simulink Converter2/LConn1 -- Transform Sensor/RConn12
  PS-Simulink Converter6/LConn1 -- Transform Sensor/RConn13
  PS-Simulink Converter3/LConn1 -- Transform Sensor/RConn14
  Transform Sensor/RConn11 -- PS-Simulink Converter4/LConn1
  Transform Sensor/RConn10 -- PS-Simulink Converter5/LConn1
  Transform Sensor/RConn9 -- PS-Simulink Converter1/LConn1
  Transform Sensor/RConn1 -- F/RConn1
  Transform Sensor/LConn1 -- B/RConn1

== system RoboticArmViperX300/vx300_base_link1 ==
  Inertia : sm_lib/Body Elements/Inertia  InertiaType=Custom  Mass=0.969034  MassUnits=kg  CenterOfMass=[0, 0, 0]  CenterOfMassUnits=m  MomentsOfInertia=[0.006024, 0.0017, 0.007162]  MomentsOfInertiaUnits=kg*m^2  ProductsOfInertia=[-8.415e-05, 3.851e-06, 4.713e-05]  ProductsOfInertiaUnits=kg*m^2  GraphicType=None  MarkerShape=Inertia  MarkerSize=20  GraphicVisPropType=SimpleVisualProperties  GraphicDiffuseColor=[0.5 0.5 0.5]  GraphicSpecularColor=[0.5 0.5 0.5 1.0]  GraphicAmbientColor=[0.15 0.15 0.15 1.0]  GraphicEmissiveColor=[0.0 0.0 0.0 1.0]  GraphicShininess=75  GraphicOpacity=1.0
  InertiaOriginTransform : sm_lib/Frames and Transforms/Rigid Transform  TranslationMethod=Cartesian  TranslationStandardOffset=0  TranslationLengthUnit=m  TranslationStandardAxis=+Z  TranslationCartesianOffset=[-0.0534774, -0.0005625750000000001, 0.0205961]  TranslationROffset=0  TranslationROffsetUnits=m  TranslationZOffset=0  TranslationZOffsetUnits=m  TranslationThetaOffset=0  TranslationThetaOffsetUnits=deg  RotationMethod=RotationSequence  RotationAngleUnits=deg  RotationStandardAxis=+Z  RotationAngle=0.0  RotationArbitraryAxis=[0 0 1]  FollAlignAxisA=+X  BaseAlignAxisA=+Y  FollAlignAxisB=+Y  BaseAlignAxisB=+Z  RotationSequenceAxes=BaseAxes  RotationSequence=XYZ  RotationSequenceAngles=[0, 0, 1.570796326794897]  RotationSequenceAnglesUnits=rad  RotationMatrix=[1 0 0; 0 1 0; 0 0 1]
  ReferenceFrame : sm_lib/Frames and Transforms/Reference Frame
  Visual : sm_lib/Body Elements/File Solid  ExtGeomFileName=ViperX_300/interbotix_xsarm_descriptions/meshes/vx300_meshes/vx300_1_base.stl  UnitType=Custom  ExtGeomFileUnits=mm  StepReaderType=HEX  ExportConvexHullGeometry=off  InertiaType=Custom  Mass=0  MassUnits=kg  CenterOfMass=[0, 0, 0]  CenterOfMassUnits=m  MomentsOfInertia=[0, 0, 0]  MomentsOfInertiaUnits=kg*m^2  ProductsOfInertia=[0, 0, 0]  ProductsOfInertiaUnits=kg*m^2  BasedOnType=DensityFromFile  Density=1000  DensityUnits=kg/m^3  DoExposeReferenceFrame=on  SerializedFrames=<Frames/>  GraphicType=FromGeometry  MarkerShape=Sphere  MarkerSize=10  GraphicVisPropType=SimpleVisualProperties  GraphicDiffuseColor=[0.5, 0.5, 0.5]  GraphicSpecularColor=[0.5 0.5 0.5 1.0]  GraphicAmbientColor=[0.15 0.15 0.15 1.0]  GraphicEmissiveColor=[0.0 0.0 0.0 1.0]  GraphicShininess=75  GraphicOpacity=1
  VisualOriginTransform : sm_lib/Frames and Transforms/Rigid Transform  TranslationMethod=Cartesian  TranslationStandardOffset=0  TranslationLengthUnit=m  TranslationStandardAxis=+Z  TranslationCartesianOffset=[0, 0, 0]  TranslationROffset=0  TranslationROffsetUnits=m  TranslationZOffset=0  TranslationZOffsetUnits=m  TranslationThetaOffset=0  TranslationThetaOffsetUnits=deg  RotationMethod=RotationSequence  RotationAngleUnits=deg  RotationStandardAxis=+Z  RotationAngle=0.0  RotationArbitraryAxis=[0 0 1]  FollAlignAxisA=+X  BaseAlignAxisA=+Y  FollAlignAxisB=+Y  BaseAlignAxisB=+Z  RotationSequenceAxes=BaseAxes  RotationSequence=XYZ  RotationSequenceAngles=[0, 0, 1.570796326794897]  RotationSequenceAnglesUnits=rad  RotationMatrix=[1 0 0; 0 1 0; 0 0 1]
  waist_AxisTransform : sm_lib/Frames and Transforms/Rigid Transform  TranslationMethod=Cartesian  TranslationStandardOffset=0  TranslationLengthUnit=m  TranslationStandardAxis=+Z  TranslationCartesianOffset=[0, 0, 0]  TranslationROffset=0  TranslationROffsetUnits=m  TranslationZOffset=0  TranslationZOffsetUnits=m  TranslationThetaOffset=0  TranslationThetaOffsetUnits=deg  RotationMethod=ArbitraryAxis  RotationAngleUnits=rad  RotationStandardAxis=+Z  RotationAngle=0  RotationArbitraryAxis=[1, 0, 0]  FollAlignAxisA=+X  BaseAlignAxisA=+Y  FollAlignAxisB=+Y  BaseAlignAxisB=+Z  RotationSequenceAxes=FollowerAxes  RotationSequence=XYX  RotationSequenceAngles=[0 0 0]  RotationSequenceAnglesUnits=deg  RotationMatrix=[1 0 0; 0 1 0; 0 0 1]
  waist_OriginTransform : sm_lib/Frames and Transforms/Rigid Transform  TranslationMethod=Cartesian  TranslationStandardOffset=0  TranslationLengthUnit=m  TranslationStandardAxis=+Z  TranslationCartesianOffset=[0, 0, 0.079]  TranslationROffset=0  TranslationROffsetUnits=m  TranslationZOffset=0  TranslationZOffsetUnits=m  TranslationThetaOffset=0  TranslationThetaOffsetUnits=deg  RotationMethod=RotationSequence  RotationAngleUnits=deg  RotationStandardAxis=+Z  RotationAngle=0.0  RotationArbitraryAxis=[0 0 1]  FollAlignAxisA=+X  BaseAlignAxisA=+Y  FollAlignAxisB=+Y  BaseAlignAxisB=+Z  RotationSequenceAxes=BaseAxes  RotationSequence=XYZ  RotationSequenceAngles=[0, 0, 0]  RotationSequenceAnglesUnits=rad  RotationMatrix=[1 0 0; 0 1 0; 0 0 1]
  F : PMIOPort  Side=Left
  F1 : PMIOPort  Port=2  Side=Right
  connections:
  waist_AxisTransform/LConn1 -- waist_OriginTransform/RConn1
  waist_AxisTransform/RConn1 -- F1/RConn1
  Visual/RConn1 -- VisualOriginTransform/RConn1
  waist_OriginTransform/LConn1 -- VisualOriginTransform/LConn1 -- InertiaOriginTransform/LConn1 -- F/RConn1 -- ReferenceFrame/RConn1
  Inertia/RConn1 -- InertiaOriginTransform/RConn1

== system RoboticArmViperX300/vx300_ee_arm_link1 ==
  Inertia : sm_lib/Body Elements/Inertia  InertiaType=Custom  Mass=0.001  MassUnits=kg  CenterOfMass=[0, 0, 0]  CenterOfMassUnits=m  MomentsOfInertia=[0.0001, 0.0001, 0.0001]  MomentsOfInertiaUnits=kg*m^2  ProductsOfInertia=[0, 0, 0]  ProductsOfInertiaUnits=kg*m^2  GraphicType=None  MarkerShape=Inertia  MarkerSize=20  GraphicVisPropType=SimpleVisualProperties  GraphicDiffuseColor=[0.5 0.5 0.5]  GraphicSpecularColor=[0.5 0.5 0.5 1.0]  GraphicAmbientColor=[0.15 0.15 0.15 1.0]  GraphicEmissiveColor=[0.0 0.0 0.0 1.0]  GraphicShininess=75  GraphicOpacity=1.0
  InertiaOriginTransform : sm_lib/Frames and Transforms/Rigid Transform  TranslationMethod=Cartesian  TranslationStandardOffset=0  TranslationLengthUnit=m  TranslationStandardAxis=+Z  TranslationCartesianOffset=[0, 0, 0]  TranslationROffset=0  TranslationROffsetUnits=m  TranslationZOffset=0  TranslationZOffsetUnits=m  TranslationThetaOffset=0  TranslationThetaOffsetUnits=deg  RotationMethod=RotationSequence  RotationAngleUnits=deg  RotationStandardAxis=+Z  RotationAngle=0.0  RotationArbitraryAxis=[0 0 1]  FollAlignAxisA=+X  BaseAlignAxisA=+Y  FollAlignAxisB=+Y  BaseAlignAxisB=+Z  RotationSequenceAxes=BaseAxes  RotationSequence=XYZ  RotationSequenceAngles=[0, 0, 0]  RotationSequenceAnglesUnits=rad  RotationMatrix=[1 0 0; 0 1 0; 0 0 1]
  ReferenceFrame : sm_lib/Frames and Transforms/Reference Frame
  gripper_AxisTransform : sm_lib/Frames and Transforms/Rigid Transform  TranslationMethod=Cartesian  TranslationStandardOffset=0  TranslationLengthUnit=m  TranslationStandardAxis=+Z  TranslationCartesianOffset=[0, 0, 0]  TranslationROffset=0  TranslationROffsetUnits=m  TranslationZOffset=0  TranslationZOffsetUnits=m  TranslationThetaOffset=0  TranslationThetaOffsetUnits=deg  RotationMethod=ArbitraryAxis  RotationAngleUnits=rad  RotationStandardAxis=+Z  RotationAngle=1.570796326794897  RotationArbitraryAxis=[-0, 1, 0]  FollAlignAxisA=+X  BaseAlignAxisA=+Y  FollAlignAxisB=+Y  BaseAlignAxisB=+Z  RotationSequenceAxes=FollowerAxes  RotationSequence=XYX  RotationSequenceAngles=[0 0 0]  RotationSequenceAnglesUnits=deg  RotationMatrix=[1 0 0; 0 1 0; 0 0 1]
  gripper_OriginTransform : sm_lib/Frames and Transforms/Rigid Transform  TranslationMethod=Cartesian  TranslationStandardOffset=0  TranslationLengthUnit=m  TranslationStandardAxis=+Z  TranslationCartesianOffset=[0.005675, 0, 0]  TranslationROffset=0  TranslationROffsetUnits=m  TranslationZOffset=0  TranslationZOffsetUnits=m  TranslationThetaOffset=0  TranslationThetaOffsetUnits=deg  RotationMethod=RotationSequence  RotationAngleUnits=deg  RotationStandardAxis=+Z  RotationAngle=0.0  RotationArbitraryAxis=[0 0 1]  FollAlignAxisA=+X  BaseAlignAxisA=+Y  FollAlignAxisB=+Y  BaseAlignAxisB=+Z  RotationSequenceAxes=BaseAxes  RotationSequence=XYZ  RotationSequenceAngles=[0, 0, 0]  RotationSequenceAnglesUnits=rad  RotationMatrix=[1 0 0; 0 1 0; 0 0 1]
  gripper_bar_OriginTransform : sm_lib/Frames and Transforms/Rigid Transform  TranslationMethod=Cartesian  TranslationStandardOffset=0  TranslationLengthUnit=m  TranslationStandardAxis=+Z  TranslationCartesianOffset=[0, 0, 0]  TranslationROffset=0  TranslationROffsetUnits=m  TranslationZOffset=0  TranslationZOffsetUnits=m  TranslationThetaOffset=0  TranslationThetaOffsetUnits=deg  RotationMethod=RotationSequence  RotationAngleUnits=deg  RotationStandardAxis=+Z  RotationAngle=0.0  RotationArbitraryAxis=[0 0 1]  FollAlignAxisA=+X  BaseAlignAxisA=+Y  FollAlignAxisB=+Y  BaseAlignAxisB=+Z  RotationSequenceAxes=BaseAxes  RotationSequence=XYZ  RotationSequenceAngles=[0, 0, 0]  RotationSequenceAnglesUnits=rad  RotationMatrix=[1 0 0; 0 1 0; 0 0 1]
  F : PMIOPort  Side=Left
  F2 : PMIOPort  Port=2  Side=Right
  F1 : PMIOPort  Port=3  Side=Right
  connections:
  gripper_bar_OriginTransform/RConn1 -- F2/RConn1
  gripper_AxisTransform/LConn1 -- gripper_OriginTransform/RConn1
  gripper_AxisTransform/RConn1 -- F1/RConn1
  gripper_bar_OriginTransform/LConn1 -- gripper_OriginTransform/LConn1 -- InertiaOriginTransform/LConn1 -- F/RConn1 -- ReferenceFrame/RConn1
  Inertia/RConn1 -- InertiaOriginTransform/RConn1

== system RoboticArmViperX300/vx300_ee_gripper_link1 ==
  Inertia : sm_lib/Body Elements/Inertia  InertiaType=Custom  Mass=0.001  MassUnits=kg  CenterOfMass=[0, 0, 0]  CenterOfMassUnits=m  MomentsOfInertia=[0.0001, 0.0001, 0.0001]  MomentsOfInertiaUnits=kg*m^2  ProductsOfInertia=[0, 0, 0]  ProductsOfInertiaUnits=kg*m^2  GraphicType=None  MarkerShape=Inertia  MarkerSize=20  GraphicVisPropType=SimpleVisualProperties  GraphicDiffuseColor=[0.5 0.5 0.5]  GraphicSpecularColor=[0.5 0.5 0.5 1.0]  GraphicAmbientColor=[0.15 0.15 0.15 1.0]  GraphicEmissiveColor=[0.0 0.0 0.0 1.0]  GraphicShininess=75  GraphicOpacity=1.0
  InertiaOriginTransform : sm_lib/Frames and Transforms/Rigid Transform  TranslationMethod=Cartesian  TranslationStandardOffset=0  TranslationLengthUnit=m  TranslationStandardAxis=+Z  TranslationCartesianOffset=[0, 0, 0]  TranslationROffset=0  TranslationROffsetUnits=m  TranslationZOffset=0  TranslationZOffsetUnits=m  TranslationThetaOffset=0  TranslationThetaOffsetUnits=deg  RotationMethod=RotationSequence  RotationAngleUnits=deg  RotationStandardAxis=+Z  RotationAngle=0.0  RotationArbitraryAxis=[0 0 1]  FollAlignAxisA=+X  BaseAlignAxisA=+Y  FollAlignAxisB=+Y  BaseAlignAxisB=+Z  RotationSequenceAxes=BaseAxes  RotationSequence=XYZ  RotationSequenceAngles=[0, 0, 0]  RotationSequenceAnglesUnits=rad  RotationMatrix=[1 0 0; 0 1 0; 0 0 1]
  ReferenceFrame : sm_lib/Frames and Transforms/Reference Frame
  F : PMIOPort  Side=Left
  connections:
  F/RConn1 -- ReferenceFrame/RConn1 -- InertiaOriginTransform/LConn1
  Inertia/RConn1 -- InertiaOriginTransform/RConn1
